simulink model "Leader"  (R2018a)
settings: Solver=FixedStepAuto  StartTime=0.0  StopTime=1000  FixedStep=0.1  RelTol=1e-3
libraries: simulink x1
settings Model: Creator=wangluo  LastModifiedBy=wangluo

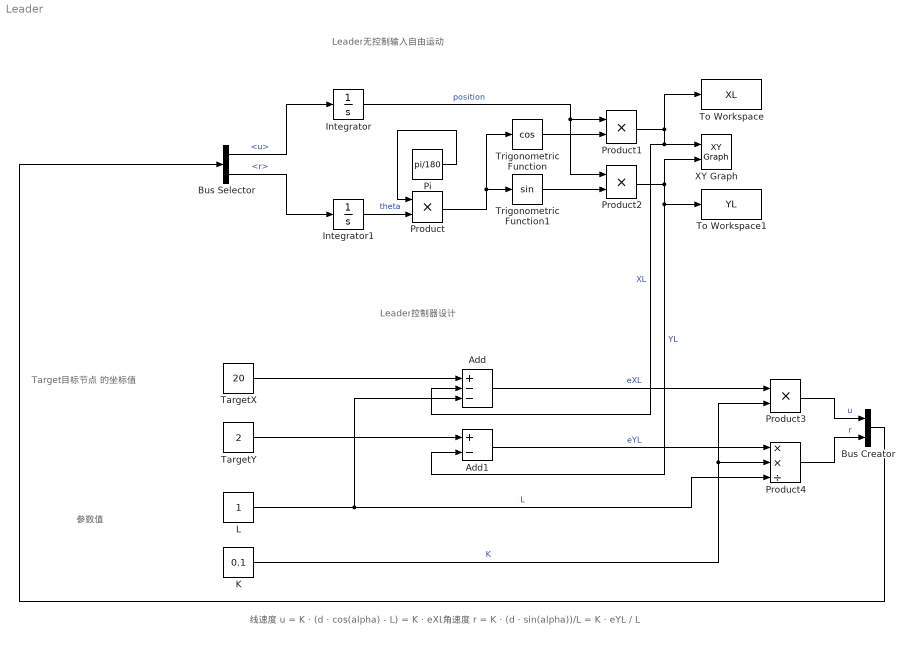
== system Leader ==
  note: Leader无控制输入自由运动
  note: Leader控制器设计
  note: Target目标节点
      | 的坐标值
  note: 参数值
  note: 线速度 u = K · (d · cos(alpha) - L) = K · eXL
      | 角速度 r = K · (d · sin(alpha))/L = K · eYL / L
  Add : Sum  Inputs=+--
  Add1 : Sum  Inputs=+-
  Bus Creator : BusCreator  Inputs=2
  Bus Selector : BusSelector  OutputSignals=u,r
  Integrator : Integrator
  Integrator1 : Integrator
  K : Constant  Value=0.1
  L : Constant
  Pi : Constant  Value=pi/180
  Product{,1..3} (4 alike) : Product
  Product4 : Product  Inputs=**/
  TargetX : Constant  Value=20
  TargetY : Constant  Value=2
  To Workspace : ToWorkspace  VariableName=XL  SaveFormat=Timeseries  SampleTime=-1
  To Workspace1 : ToWorkspace  VariableName=YL  SaveFormat=Timeseries  SampleTime=-1
  Trigonometric Function : Trigonometry  Operator=cos
  Trigonometric Function1 : Trigonometry
  XY Graph : simulink/Sinks/XY Graph  xmin=-20  xmax=50  ymin=-20  ymax=50  st=-1
  wires:
  Integrator1/1 -> Product/2  "theta"
  Pi/1 -> Product/1
  Product1/1 -> To Workspace/1, XY Graph/1, Add/2  "XL"
  Product2/1 -> XY Graph/2, Add1/2, To Workspace1/1  "YL"
  Trigonometric Function/1 -> Product1/2
  Trigonometric Function1/1 -> Product2/2
  Integrator/1 -> Product2/1, Product1/1  "position"
  Product/1 -> Trigonometric Function1/1, Trigonometric Function/1
  TargetX/1 -> Add/1
  TargetY/1 -> Add1/1
  Add/1 -> Product3/1  "eXL"
  Add1/1 -> Product4/1  "eYL"
  L/1 -> Product4/3, Add/3  "L"
  K/1 -> Product4/2, Product3/2  "K"
  Product4/1 -> Bus Creator/2  "r"
  Product3/1 -> Bus Creator/1  "u"
  Bus Creator/1 -> Bus Selector/1
  Bus Selector/1 -> Integrator/1  "<u>"
  Bus Selector/2 -> Integrator1/1  "<r>"
